simulink model "pure_pursuit_20b"  (R2020b)
settings: Solver=FixedStepAuto  StartTime=0.0  StopTime=1000  FixedStep=0.01  RelTol=1e-3
values from neighbouring files (symbols this model uses):
  path = [0 14.78 15.6427 16 16 15.6427 14.78 1.22 0.3573 0 0 0.3573 ... (52 elements, 26x2)]    [finalGrass.mat]    (also in parking_lot_paper1.mat; prerun.m = waypoints)
  speed = 2    [finalGrass.mat]    (also in parking_lot_paper1.mat; prerun.m)
undefined symbols (not defined in the file or in its folder): Angular, Linear
libraries: robotlib x3, robotalgslib x1, fuzblock x1, simulink x1
settings Model: Creator=dev  LastModifiedBy=dev
settings DataIOCC: SaveFormat=Array  ReturnWorkspaceOutputs=off
settings OptimizationCC: EnhancedBackFolding=on  PassReuseOutputArgsThreshold=0  MaxStackSize=64  OptimizeBlockOrder=speed  DifferentSizesBufferReuse=on  OptimizationCustomize=off
settings DebuggingCC: ParameterTunabilityLossMsg=error
settings HardwareCC: ProdBitPerPointer=32  ProdBitPerSizeT=32  ProdBitPerPtrDiffT=32  ProdLargestAtomicFloat=None  ProdIntDivRoundTo=Undefined  ProdEndianess=Unspecified  ProdWordSize=32  ProdHWDeviceType=Generic->Unspecified (assume 32-bit Generic)  UseEmbeddedCoderFeatures=off
settings SFSimCC: MATLABDynamicMemAlloc=off  CustomCodeUndefinedFunction=UseInterfaceOnly  SimTargetLang=C++
settings RTWCC: Description=Embedded Coder  SystemTargetFile=ert.tlc  HardwareBoard=Robot Operating System (ROS)  TLCOptions="-aInlineSetEventsForThisBaseRateFcn=TLC_FALSE -aSuppressMultiTaskScheduler=TLC_FALSE  -aRateBasedStepFcn=0"  TemplateMakefile=ert_default_tmf  GenerateReport=on  Toolchain=Catkin  LaunchReport=on  TargetLang=C++
settings CodeAppCC: ForceParamTrailComments=on  OperatorAnnotations=on
settings ERTTargetCC: ERTCustomFileBanners=off  SupportContinuousTime=on  SupportNonInlinedSFcns=on  RemoveResetFunc=off  ModelStepFunctionPrototypeControlCompliant=off

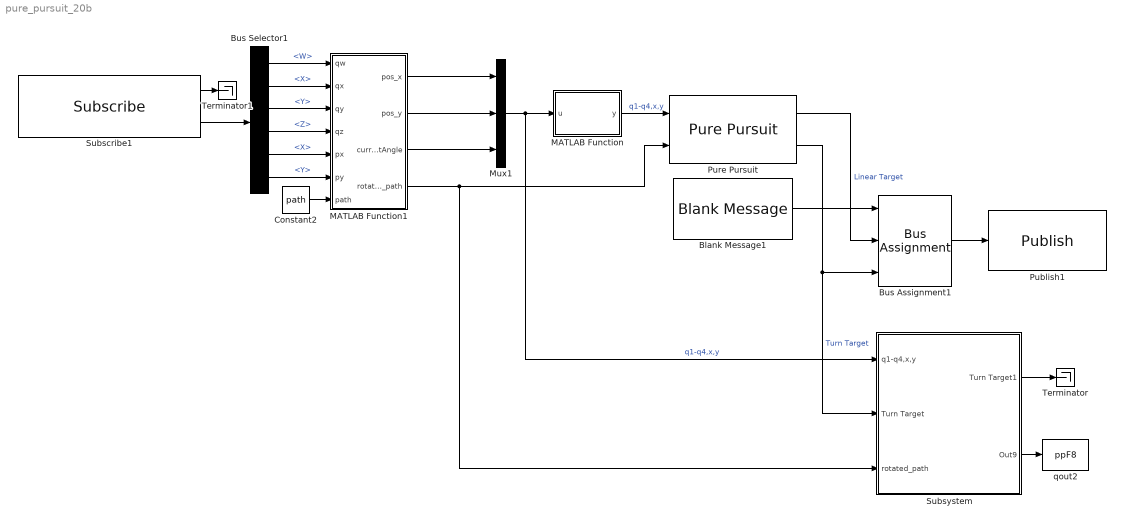
== system pure_pursuit_20b ==
  Blank Message1 : robotlib/Blank Message  messageClass=Message  entityType=geometry_msgs/Twist  messageType=geometry_msgs/Twist  SampleTime=inf  legacyBusStruct=off
  Bus Assignment1 : BusAssignment  AssignedSignals=Linear.X,Angular.Z
  Bus Selector1 : BusSelector  OutputSignals=Pose.Pose.Orientation.W,Pose.Pose.Orientation.X,Pose.Pose.Orientation.Y,Pose.Pose.Orientation.Z,Pose.Pose.Position.X,Pose.Pose.Position.Y
  Constant2 : Constant  Value=path
  MATLAB Function : MATLAB Function  TreatAsAtomicUnit=on
  MATLAB Function1 : MATLAB Function  TreatAsAtomicUnit=on
  Mux1 : Mux  Inputs=3
  Publish1 : robotlib/Publish  topicSource=Select from ROS network  topic=/cmd_vel  messageType=geometry_msgs/Twist  legacyBusStruct=off  messageQueueLength=1
  Pure Pursuit : robotalgslib/Pure Pursuit  DesiredLinearVelocity=speed  MaxAngularVelocity=angVeloSat  LookaheadDistance=lookahead  TargetDirPort=off  SimulateUsing=Interpreted execution
  Subscribe1 : robotlib/Subscribe  topicSource=Select from ROS network  topic=/odometry/filtered  messageType=nav_msgs/Odometry  SampleTime=-1  legacyBusStruct=off  messageQueueLength=1
  Subsystem : Subsystem
  Terminator : Terminator
  Terminator1 : Terminator
  qout2 : ToWorkspace  VariableName=ppF8  SampleTime=-1
  wires:
  Subscribe1/2 -> Bus Selector1/1
  Pure Pursuit/1 -> Bus Assignment1/2  "Linear Target"
  Bus Assignment1/1 -> Publish1/1
  Blank Message1/1 -> Bus Assignment1/1
  MATLAB Function1/4(rotated_path) -> Subsystem/3(rotated_path), Pure Pursuit/2
  MATLAB Function/1(y) -> Pure Pursuit/1  "q1-q4,x,y"
  Pure Pursuit/2 -> Subsystem/2(Turn Target), Bus Assignment1/3  "Turn Target"
  Mux1/1 -> MATLAB Function/1(u), Subsystem/1(q1-q4,x,y)  "q1-q4,x,y"
  Subsystem/2(Out9) -> qout2/1
  Subsystem/1(Turn Target1) -> Terminator/1
  Bus Selector1/1 -> MATLAB Function1/1(qw)  "<W>"
  Bus Selector1/2 -> MATLAB Function1/2(qx)  "<X>"
  Bus Selector1/3 -> MATLAB Function1/3(qy)  "<Y>"
  Bus Selector1/4 -> MATLAB Function1/4(qz)  "<Z>"
  Bus Selector1/5 -> MATLAB Function1/5(px)  "<X>"
  Bus Selector1/6 -> MATLAB Function1/6(py)  "<Y>"
  Constant2/1 -> MATLAB Function1/7(path)
  MATLAB Function1/2(pos_y) -> Mux1/2
  MATLAB Function1/1(pos_x) -> Mux1/1
  MATLAB Function1/3(currentAngle) -> Mux1/3
  Subscribe1/1 -> Terminator1/1

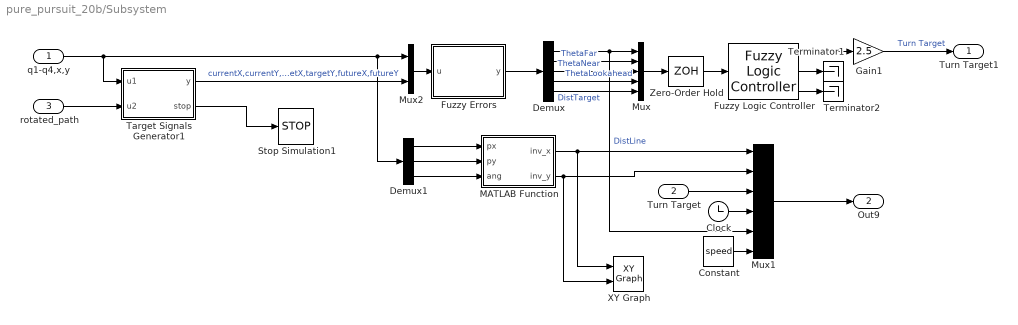
== system pure_pursuit_20b/Subsystem ==
  q1-q4,x,y : Inport
  Turn Target : Inport  Port=2
  rotated_path : Inport  Port=3
  Clock : Clock
  Constant : Constant  Value=speed
  Demux : Demux  Outputs=5
  Demux1 : Demux  Outputs=3
  Fuzzy Errors : MATLAB Function  TreatAsAtomicUnit=on
  Fuzzy Logic Controller : fuzblock/Fuzzy Logic  Controller  FIS='fuzzyControl.fis'  OutputSampleNumber=3000  DataType=double  FuzzifiedInputs=off  RuleFiringStrengths=on  RuleOutputs=off  AggregatedOutputs=on  SimulateUsing=Code generation  OutOfRangeInputValueMessage=warning  NoRuleFiredMessage=warning  EmptyOutputFuzzySetMessage=warning
  Gain1 : Gain  Gain=2.5
  MATLAB Function : MATLAB Function  TreatAsAtomicUnit=on
  Mux : Mux  Inputs=5
  Mux1 : Mux  Inputs=6
  Mux2 : Mux  Inputs=2
  Stop Simulation1 : Stop
  Target Signals Generator1 : MATLAB Function  TreatAsAtomicUnit=on
  Terminator1 : Terminator
  Terminator2 : Terminator
  XY Graph : simulink/Sinks/XY Graph  xmin=-10  xmax=10  ymin=-10  ymax=10  st=-1
  Zero-Order Hold : ZeroOrderHold  SampleTime=.01
  Turn Target1 : Outport
  Out9 : Outport  Port=2
  wires:
  Demux/3 -> Mux/3  "ThetaNear"
  Target Signals Generator1/1(y) -> Mux2/2  "currentX,currentY,targetX,targetY,futureX,futureY"
  Turn Target/1 -> Mux1/3
  Mux1/1 -> Out9/1
  Fuzzy Errors/1(y) -> Demux/1
  q1-q4,x,y/1 -> Demux1/1, Mux2/1, Target Signals Generator1/1(u1)
  Gain1/1 -> Turn Target1/1  "Turn Target"
  Fuzzy Logic Controller/1 -> Gain1/1
  Demux/5 -> Mux/5  "DistTarget"
  Target Signals Generator1/2(stop) -> Stop Simulation1/1
  Demux1/3 -> MATLAB Function/3(ang)
  Mux2/1 -> Fuzzy Errors/1(u)
  Mux/1 -> Zero-Order Hold/1
  Demux/2 -> Mux/2  "ThetaFar"
  rotated_path/1 -> Target Signals Generator1/2(u2)
  Clock/1 -> Mux1/4
  Zero-Order Hold/1 -> Fuzzy Logic Controller/1
  Demux/1 -> Mux/1, Mux1/5  "DistLine"
  Demux/4 -> Mux/4  "ThetaLookahead"
  Constant/1 -> Mux1/6
  Fuzzy Logic Controller/2 -> Terminator1/1
  Fuzzy Logic Controller/3 -> Terminator2/1
  Demux1/2 -> MATLAB Function/2(py)
  Demux1/1 -> MATLAB Function/1(px)
  MATLAB Function/1(inv_x) -> XY Graph/1, Mux1/1
  MATLAB Function/2(inv_y) -> XY Graph/2, Mux1/2

== matlab function pure_pursuit_20b/MATLAB Function1 ==
  data: pos_x output; pos_y output; qw input; currentAngle output; qx input; qy input; qz input; px input; py input; path input; rotated_path output
function [pos_x, pos_y, currentAngle, rotated_path] = fcn(qw, qx, qy, qz, px, py, path)
    persistent init_x;
    persistent init_y;
    persistent init_ang;
    persistent rotation;
    if isempty(init_x)
        init_x = px;
        init_y = py;
        init_ang = -atan2(2*(qw*qz + qx*qy),1-2*(qy^2 + qz^2));
        if((init_ang < -pi) || (pi < init_ang))
            init_ang = mod(init_ang+pi, 2*pi)-pi;
        end
        rotation = [cos(init_ang), -sin(init_ang);
            sin(init_ang),  cos(init_ang)];
    end
    pos_x = px - init_x;
    pos_y = py - init_y;
    currentAngle = atan2(2*(qw*qz + qx*qy),1-2*(qy^2 + qz^2));
    if((currentAngle < -pi) || (pi < currentAngle))
        currentAngle = mod(currentAngle+pi, 2*pi)-pi;
    end
    rotated_path = path * rotation; 
end

== matlab function pure_pursuit_20b/MATLAB Function ==
  data: u input; y output
function y = fcn(u)
    y = [u(1), u(2), u(3)];
end

== matlab function pure_pursuit_20b/Subsystem/Target Signals Generator1 ==
  data: u1 input; y output; u2 input; stop output
function [y,stop] = fcn(u1,u2)
persistent pathcount;
persistent pathlength;
persistent path; %error in code, initially used path but this is already a matlab function
persistent pathPre;

if isempty(pathcount)
   pathcount=1;
   pathPre=u2;
   [pathlength,~]=size(pathPre);  
   path=[pathPre; pathPre(pathlength,1)+100 pathPre(pathlength,2)+100]; %sim takes multiple iterations to stop after reaching final point, so this prevents it from breaking
end

pos=[u1(1), u1(2)]; % [x,y] 
currentPoint=path(pathcount,:);
target=path(pathcount+1,:);

A = [(currentPoint(2)-target(2)), target(1)-currentPoint(1); target(1)-currentPoint(1), target(2)-currentPoint(2)];
b = [ target(1)*currentPoint(2)-currentPoint(1)*target(2); pos(1)*(target(1)-currentPoint(1)) + pos(2)*(target(2)-currentPoint(2))];
proj = (A\b)'; %projected point on the line between  .
projLen=dot(proj-currentPoint,target-currentPoint)/norm(target-currentPoint)^2; %the distance along the projected line, where 0 is the start point and 1 is the end point

if ((projLen>1))
    pathcount=pathcount+1;
end

%check if at destination and terminate sim if there
pathflag=0;
if (pathcount==pathlength)
    pathflag=1;
end

if ((pathcount==(pathlength-1))||(pathcount==(pathlength)))
    a=path(pathcount,:);
    b=path(pathcount+1,:);
    diff = (b-a) / norm(b-a);
    post = b + diff;
else
    a=path(pathcount,:);
    b=path(pathcount+1,:);
    post=path(pathcount+2,:);
end

y = [a(1);a(2);b(1);b(2);post(1);post(2)];
stop=pathflag;

== matlab function pure_pursuit_20b/Subsystem/MATLAB Function ==
  data: px input; inv_x output; py input; ang input; inv_y output
function [inv_x, inv_y] = fcn(px, py, ang)
    persistent init_ang;
    persistent rotation_inv;
    if isempty(init_ang)
        init_ang = -ang;
        rotation_inv = [cos(init_ang), sin(init_ang);
                       -sin(init_ang),  cos(init_ang)];
    end
    rotated_path = [px,py] * rotation_inv;
    inv_x = rotated_path(1);
    inv_y = rotated_path(2);
end

== matlab function pure_pursuit_20b/Subsystem/Fuzzy Errors ==
  settings: updateMethod=DISCRETE
  data: u input; y output
function y  = fcn(u)
kLOOK = 0.95;

pos=[u(1), u(2)]; % [x,y]
currentAngle=u(3);

currentPoint=[u(4) u(5)];
target=[u(6) u(7)];
future=[u(8) u(9)];

A = [(currentPoint(2)-target(2)), target(1)-currentPoint(1); target(1)-currentPoint(1), target(2)-currentPoint(2)];
b = [ target(1)*currentPoint(2)-currentPoint(1)*target(2); pos(1)*(target(1)-currentPoint(1)) + pos(2)*(target(2)-currentPoint(2))];
proj = (A\b)'; %projected point on the line between  .

d = ( pos(1)-currentPoint(1) )*(target(2)-currentPoint(2)) - (pos(2)-currentPoint(2))*(target(1)-currentPoint(1));

if ( d >0)
    side = 1;
elseif ( d < 0)
    side = -1;
else
    side = 0;
end

distanceLine=norm(pos-proj)*side;
distanceTarget=sqrt((target(1)-pos(1))^2+(target(2)-pos(2))^2);

%wrap to +/-pi
if((currentAngle < -pi) || (pi < currentAngle))
    currentAngle = mod(currentAngle+pi, 2*pi)-pi;
end

farTarget=[kLOOK*proj(1)+(1-kLOOK)*target(1) kLOOK*proj(2)+(1-kLOOK)*target(2)];

th1 = atan2(farTarget(2)-pos(2), farTarget(1)-pos(1));
th2 = atan2(target(2)-currentPoint(2), target(1)-currentPoint(1));
th3 = atan2(future(2)-target(2), future(1)-target(1)); 

ThetaFar=th1-currentAngle;
ThetaNear=th2-currentAngle;
ThetaLookahead=th3-currentAngle;

%wrap to +/-pi
if((ThetaFar < -pi) || (pi < ThetaFar))
    ThetaFar = mod(ThetaFar+pi, 2*pi)-pi;
end

%wrap to +/-pi
if((ThetaNear < -pi) || (pi < ThetaNear))
    ThetaNear = mod(ThetaNear+pi, 2*pi)-pi;
end

%wrap to +/-pi
if((ThetaLookahead < -pi) || (pi < ThetaLookahead))
    ThetaLookahead = mod(ThetaLookahead+pi, 2*pi)-pi;
end

y = [distanceLine;ThetaFar;ThetaNear;ThetaLookahead;distanceTarget];
